simulink model "MPC_Final"  (R2025b)
settings: Solver=ode4  StartTime=0.0  StopTime=10  FixedStep=0.005  RelTol=1e-3  EnableMultiTasking=on
settings Model: Creator=nabil  LastModifiedBy=Mohamed Reda
settings SolverCC: PositivePriorityOrder=on
settings DataIOCC: SaveOutput=off  SaveTime=off
settings OptimizationCC: DefaultParameterBehavior=Inlined  StrengthReduction=on  PassReuseOutputArgsAs=Individual arguments  ZeroExternalMemoryAtStartup=off  ZeroInternalMemoryAtStartup=off  MaxStackSize=200000  OptimizeBlockOrder=speed  OptimizationPriority=Speed  OptimizationCustomize=off  MultiThreadedLoops=on  AutoScheduleForLoops=on  EfficientTunableParamExpr=on
settings DebuggingCC: ParameterTunabilityLossMsg=error
settings HardwareCC: ProdBitPerLong=64.0  ProdBitPerPtrDiffT=32.0  ProdLargestAtomicFloat=None  ProdHWDeviceType=Custom Processor->Custom Processor
settings SFSimCC: SimUserIncludeDirs=./Simulation_ert_rtw/
settings SFSimCC: SimUserSources=|
  | functions.c
  | Simulation.c
  | Simulation_data.c
settings RTWCC: SystemTargetFile=ert.tlc  TemplateMakefile=ert_default_tmf  CustomInclude=./Simulation_ert_rtw/  BuildConfiguration=Faster Runs  Description=Embedded Coder
settings RTWCC: CustomHeaderCode=|
  | functions.h
  | Simulation.h
settings RTWCC: CustomSource=|
  | functions.c
  | Simulation.c
settings CodeAppCC: ForceParamTrailComments=on  IgnoreCustomStorageClasses=off  OperatorAnnotations=on  SimulinkDataObjDesc=on  SFDataObjDesc=on  InsertBlockDesc=on
settings ERTTargetCC: ExtModeTransport=2.0  ExtModeStaticAlloc=on  ExtModeMexFile=ext_xcp  ExtModeIntrfLevel=Level2 - Open  ERTCustomFileTemplate=example_file_process.tlc  SupportNonFinite=off  SupportVariableSizeSignals=on

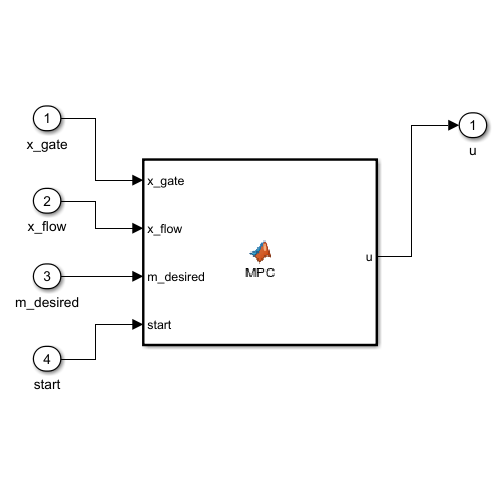
[thumbnail: Simulink's stored preview of the top-level diagram]
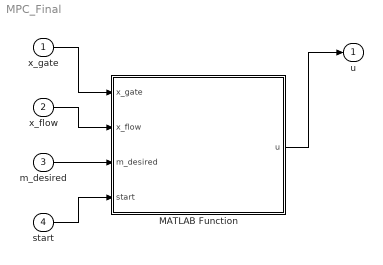
== system MPC_Final ==
  x_gate : Inport  OutDataTypeStr=double  PortDimensions=7  SampleTime=[0.0050000000000000001,0]
  x_flow : Inport  Port=2  OutDataTypeStr=double  PortDimensions=9  SampleTime=[0.0050000000000000001,0]
  m_desired : Inport  Port=3  OutDataTypeStr=double  PortDimensions=1  SampleTime=[0.0050000000000000001,0]
  start : Inport  Port=4  OutDataTypeStr=double  PortDimensions=1  SampleTime=[0.0050000000000000001,0]
  MATLAB Function : MATLAB Function  TreatAsAtomicUnit=on
  u : Outport  OutDataTypeStr=double  PortDimensions=1  SampleTime=[0.0050000000000000001,0]
  wires:
  x_gate/1 -> MATLAB Function/1(x_gate)
  x_flow/1 -> MATLAB Function/2(x_flow)
  m_desired/1 -> MATLAB Function/3(m_desired)
  start/1 -> MATLAB Function/4(start)
  MATLAB Function/1(u) -> u/1

== matlab function MPC_Final/MATLAB Function ==
  data: x_gate input; u output; x_flow input; m_desired input; start input
function u  = MPC(x_gate,x_flow,m_desired,start)
u=0;
[u] = NMPC(x_gate,x_flow,m_desired,start);
